simulink model "AV_7_ZADACA2_shpic_vo_D_komponenta"  (R2018a)
settings: Solver=VariableStepAuto  StartTime=0.0  StopTime=2500  RelTol=1e-3
libraries: simulink_extras x2
settings Model: Creator=DD  LastModifiedBy=DD

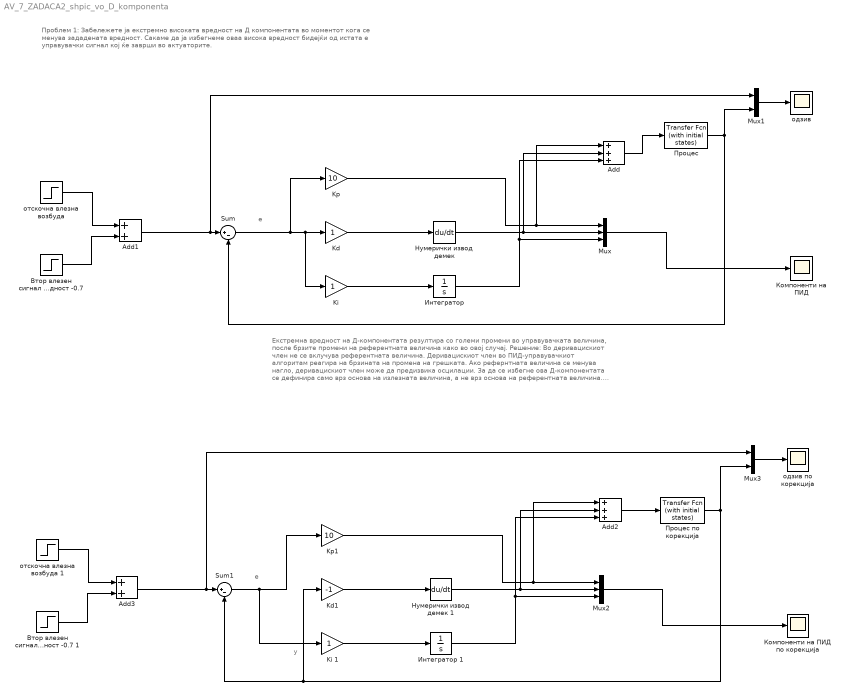
== system AV_7_ZADACA2_shpic_vo_D_komponenta ==
  note: у
  note: Екстремна вредност на Д-компонентата резултира со големи промени во управувачката величина, после брзите промени на референтната величина како во овој случај. Решение: Во деривацискиот член не се вклучува референтната величина. Деривацискиот член во ПИД-управувачкиот алгоритам реагира на брзината на промена на грешката. Ако рефернтната величина се менува нагло, деривацискиот член може да предизвика осцилации. За да се избегне ова Д-компонентата се дефинира само врз основа на излезната величина, а не врз основа на референтната величина. Овие модифицирани алгоритми се помалку чувствителни на високо-фреквентни сигнали на референтната величина, отколки на тие од излезната величина. Ова значи дека овој модификуван ПИД повеќе реагира на излезниот сигнал, отколку на референтниот сигнал. Ако референтната величина има брзи фреквентни промени, алгоритмот не реагира агресивно на нив. Но, ако излезниот сигнал има брзи промени, алгоритмот ќе ги следи и реагира на нив.
      | Поглавје VI-3.3
  note: е
  note: Проблем 1: Забележете ја екстремно високата вредност на Д компонентата во моментот кога се менува зададената вредност. Сакаме да ја избегнеме оваа висока вредност бидејќи од истата е управувачки сигнал кој ќе заврши во актуаторите.
  note: е
  Add : Sum  Inputs=+++
  Add1 : Sum
  Add2 : Sum  Inputs=+++
  Add3 : Sum
  Kd : Gain
  Kd1 : Gain  Gain=-1
  "Ki " : Gain
  Ki 1 : Gain
  Kp : Gain  Gain=10
  Kp1 : Gain  Gain=10
  Mux : Mux  Inputs=3
  Mux1 : Mux  Inputs=2
  Mux2 : Mux  Inputs=3
  Mux3 : Mux  Inputs=2
  Sum : Sum  Inputs=|+-
  Sum1 : Sum  Inputs=|+-
  "Втор влезен сигнал со крајна вредност -0.7 " : Step  Time=300  After=-0.7  SampleTime=0
  Втор влезен сигнал со крајна вредност -0.7 1 : Step  Time=300  After=-0.7  SampleTime=0
  "Интегратор " : Integrator
  Интегратор 1 : Integrator
  Компоненти на ПИД : Scope
  Компоненти на ПИД по корекција : Scope
  "Нумерички извод демек " : Derivative
  Нумерички извод демек 1 : Derivative
  "Процес " : simulink_extras/Additional Linear/Transfer Fcn (with initial states)  N=[1]  D="[1  10 20]"  X0=0.1
  Процес по корекција : simulink_extras/Additional Linear/Transfer Fcn (with initial states)  N=[1]  D="[1  10 20]"  X0=0.1
  одзив : Scope
  одзив по корекција : Scope
  "отскочна влезна возбуда " : Step  Time=0  SampleTime=0
  отскочна влезна возбуда 1 : Step  Time=0  SampleTime=0
  wires:
  Mux1/1 -> одзив/1
  "Нумерички извод демек "/1 -> Mux/2, Add/2
  Mux/1 -> Компоненти на ПИД/1
  "Процес "/1 -> Sum/2, Mux1/2
  Add/1 -> "Процес "/1
  Kd/1 -> "Нумерички извод демек "/1
  "Интегратор "/1 -> Mux/3, Add/3
  "Ki "/1 -> "Интегратор "/1
  Sum/1 -> Kp/1, "Ki "/1, Kd/1
  Kp/1 -> Mux/1, Add/1
  "отскочна влезна возбуда "/1 -> Add1/1
  Add1/1 -> Mux1/1, Sum/1
  "Втор влезен сигнал со крајна вредност -0.7 "/1 -> Add1/2
  Sum1/1 -> Ki 1/1, Kp1/1
  Kp1/1 -> Mux2/1, Add2/1
  Add2/1 -> Процес по корекција/1
  Mux2/1 -> Компоненти на ПИД по корекција/1
  Kd1/1 -> Нумерички извод демек 1/1
  Процес по корекција/1 -> Mux3/2, Kd1/1, Sum1/2
  Интегратор 1/1 -> Mux2/3, Add2/3
  Mux3/1 -> одзив по корекција/1
  отскочна влезна возбуда 1/1 -> Add3/1
  Ki 1/1 -> Интегратор 1/1
  Втор влезен сигнал со крајна вредност -0.7 1/1 -> Add3/2
  Add3/1 -> Mux3/1, Sum1/1
  Нумерички извод демек 1/1 -> Mux2/2, Add2/2
